simulink model "test1"  (R2018a)
settings: Solver=VariableStepAuto  StartTime=0.0  StopTime=4000  FixedStep=0.01  RelTol=1e-3
InitFcn:
  | run constants
StopFcn:
  | run runafter
values from neighbouring files (symbols this model uses):
  F_0 = [0 0 0]    [constants2.m]
  F_grav = mass_0 * g_h    (= 7.95745129095)    [constants2.m]
  phi_noise = noise_att_on * noise_att_mag    [constants2.m]
  pm_0 = [0 0 0]    [constants2.m]
  Psi_noise = noise_att_on * noise_att_mag    [constants2.m]
  T_d = Td_on * [0.001 0.001 0.001]    [constants2.m]
  theta_noise = noise_att_on * noise_att_mag    [constants2.m]
  Vm_0 = [0 Vc 0]    [constants2.m]
  xme_0 = [1 2 3]    [constants2.m]
libraries: shared6dof x6, simulink x4, shared6dofsys x3, sharedutil x1, dspmathops x1
CloseFcn:
  | run runafter
settings Model: EnablePacing=on  PacingRate=1000  Creator=Matt  LastModifiedBy=matth

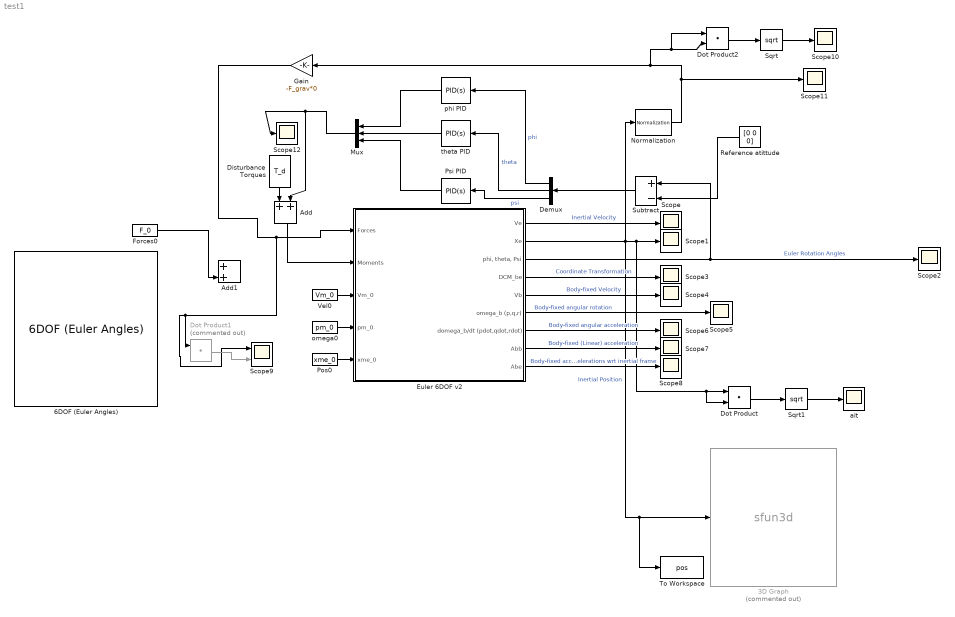
== system test1 ==
  3D Graph : S-Function  Commented=on  LoadFcn=if exist('sfun3d','file'), sfun3d([],[],[],'LoadBlock'); end  FunctionName=sfun3d  Parameters=ax,T,np,cp,gd,ls,mk,mx,hd,tb  SFunctionDeploymentMode=off  EnableBusSupport=off  mask(3D Graph){np=1, ax=[-3 3 -3 3 -3 3], mx=1e4, T=0.1, cp=[3 2 1], gd=on, hd=off, tb=off, ls=-, mk=none}
      mask prompts: np "Number of moving points (lines)"; ax "Range: [xmin xmax  ymin ymax zmin zmax]"; mx "Max number of points in each line"; T "Sampling Time"; cp "Camera position (use [0 0 1] for 2D XY view)"; gd "Grid (on|off)"; hd "HeadMarkers (on|off)"; tb "Toolbar (on|off)"; ls "LineStyle"; mk "LineMarker"
      mask help:
      | This block plots the position of several points in the XYZ space. The input contains the coordinates of all the points (x1,y1,z1,x2,y2,z2,...).
      | The number of moving points (lines), the XYZ ranges, sampling time, camera position, and grid (among other things) can be set as mask parameters.
      settings: CopyFcn=if exist('sfun3d','file'), sfun3d([],[],[],'CopyBlock'); end  DeleteFcn=if exist('sfun3d','file'), sfun3d([],[],[],'DeleteBlock'); end  NameChangeFcn=if exist('sfun3d','file'), sfun3d([],[],[],'NameChange'); end
      mask Help:
      | This block plots the position of several points in the XYZ space. The input contains the coordinates of all the points (x1,y1,z1,x2,y2,z2,...).
      | The number of moving points (lines), the XYZ ranges, sampling time, camera position, and grid (among other things) can be set as mask parameters.
      mask TypeOptions ls: - | -- | : | -. | none
      mask TypeOptions mk: none | . | + | o | * | x | square | diamond | v | ^ | > | < | pentagram | hexagram
      mask Display: plot([.05 .95 .95 .05 .05],[.45 .45 .95 .95 .45], 0.5+cos(0:0.1:2*pi)*0.3,0.7+sin(0:0.1:2*pi)*0.2)
  6DOF (Euler Angles) : shared6dof/6DOF (Euler Angles)  units=Metric (MKS)  mtype=Fixed  rep=Euler Angles  xme_0=[0 0 0]  Vm_0=[0 0 0]  eul_0=[0 0 0]  pm_0=[0 0 0]  mass_0=1.0  mass_e=0.5  mass_f=2.0  inertia=eye(3)  inertia_e=eye(3)  inertia_f=2*eye(3)  k_quat=1.0  vre_flag=on  abi_flag=off  aMode=0
      settings: SourceProductBaseCode=AE
  Add : Sum
  Add1 : Sum
  Demux : Demux  Outputs=3
  Disturbance Torques : Constant  Value=T_d
  Dot Product : DotProduct  InputSameDT=on  OutDataTypeStr=Inherit: Inherit via internal rule
  Dot Product1 : DotProduct  Commented=on  InputSameDT=on  OutDataTypeStr=Inherit: Inherit via internal rule
  Dot Product2 : DotProduct  InputSameDT=on  OutDataTypeStr=Inherit: Inherit via internal rule
  Euler 6DOF v2 : Subsystem
  Forces0 : Constant  Value=F_0
  Gain : Gain  Gain=-F_grav*0
  Mux : Mux  Inputs=3
  Normalization : dspmathops/Normalization  NormType=2-norm  Bias=1e-10  NormOver=Each column  Dimension=1  roundingMode=Floor  overflowMode=off  accumDataTypeStr=Inherit: Same as product output  accumLastDataTypeStr=Inherit: Same as product output  outputDataTypeStr=Inherit: Same as product output  outputMin=[]  outputMax=[]  outputLastDataTypeStr=Inherit: Same as product output
      settings: SourceProductName=DSP System Toolbox
  Pos0 : Constant  Value=xme_0
  Psi PID : simulink/Continuous/PID Controller  Controller=PID  TimeDomain=Continuous-time  SampleTime=-1  IntegratorMethod=Forward Euler  FilterMethod=Forward Euler  Form=Parallel  UseFilter=on  ControllerParametersSource=internal  P=-730.157338378478  I=-36.609264068618  D=-2842.71233291057  N=10.4897155810233  InitialConditionSource=internal  InitialConditionForIntegrator=0  InitialConditionForFilter=0  ExternalReset=none  LimitOutput=off  UpperSaturationLimit=inf  LowerSaturationLimit=-inf  LinearizeAsGain=on  AntiWindupMode=none  Kb=1  TrackingMode=off  Kt=1  PParamMin=[]  PParamMax=[]  IParamMin=[]  IParamMax=[]  DParamMin=[]  DParamMax=[]  NParamMin=[]  NParamMax=[]  KbParamMin=[]  KbParamMax=[]  KtParamMin=[]  KtParamMax=[]  POutMin=[]  POutMax=[]  IOutMin=[]  IOutMax=[]  DOutMin=[]  DOutMax=[]  NOutMin=[]  NOutMax=[]  KbOutMin=[]  KbOutMax=[]  KtOutMin=[]  KtOutMax=[]  IntegratorOutMin=[]  IntegratorOutMax=[]  FilterOutMin=[]  FilterOutMax=[]  SumOutMin=[]  SumOutMax=[]  SumI1OutMin=[]  SumI1OutMax=[]  SumI2OutMin=[]  SumI2OutMax=[]  SumI3OutMin=[]  SumI3OutMax=[]  SumDOutMin=[]  SumDOutMax=[]  SaturationOutMin=[]  SaturationOutMax=[]  IntegratorContinuousStateAttributes=''  IntegratorStateMustResolveToSignalObject=off  IntegratorRTWStateStorageClass=Auto  FilterContinuousStateAttributes=''  FilterStateMustResolveToSignalObject=off  FilterRTWStateStorageClass=Auto  DifferentiatorICPrevScaledInput=0  DifferentiatorOutMin=[]  DifferentiatorOutMax=[]  FilterDiffOutCoefMin=[]  FilterDiffOutCoefMax=[]  SumDenOutMin=[]  SumDenOutMax=[]  SumNumOutMin=[]  SumNumOutMax=[]  ReciprocalOutMin=[]  ReciprocalOutMax=[]  DivideOutMin=[]  DivideOutMax=[]  TunerSelectOption=Transfer Function Based (PID Tuner App)
  Reference atittude : Constant  Value=[0 0 0]
  Scope{,1..8,10..12} (12 alike) : Scope
  Scope9 : Scope  NumInputPorts=2
  Sqrt : Sqrt  SaturateOnIntegerOverflow=on
  Sqrt1 : Sqrt  SaturateOnIntegerOverflow=on
  Subtract : Sum  Inputs=+-
  To Workspace : ToWorkspace  VariableName=pos  SaveFormat=Timeseries  SampleTime=-1
  Vel0 : Constant  Value=Vm_0
  alt : Scope
  "omega0 " : Constant  Value=pm_0
  "phi PID " : simulink/Continuous/PID Controller  Controller=PID  TimeDomain=Continuous-time  SampleTime=-1  IntegratorMethod=Forward Euler  FilterMethod=Forward Euler  Form=Parallel  UseFilter=on  ControllerParametersSource=internal  P=-464.198158177747  I=-21.7313338529705  D=-2434.80245399495  N=5.45397025421619  InitialConditionSource=internal  InitialConditionForIntegrator=0  InitialConditionForFilter=0  ExternalReset=none  LimitOutput=off  UpperSaturationLimit=inf  LowerSaturationLimit=-inf  LinearizeAsGain=on  AntiWindupMode=none  Kb=1  TrackingMode=off  Kt=1  PParamMin=[]  PParamMax=[]  IParamMin=[]  IParamMax=[]  DParamMin=[]  DParamMax=[]  NParamMin=[]  NParamMax=[]  KbParamMin=[]  KbParamMax=[]  KtParamMin=[]  KtParamMax=[]  POutMin=[]  POutMax=[]  IOutMin=[]  IOutMax=[]  DOutMin=[]  DOutMax=[]  NOutMin=[]  NOutMax=[]  KbOutMin=[]  KbOutMax=[]  KtOutMin=[]  KtOutMax=[]  IntegratorOutMin=[]  IntegratorOutMax=[]  FilterOutMin=[]  FilterOutMax=[]  SumOutMin=[]  SumOutMax=[]  SumI1OutMin=[]  SumI1OutMax=[]  SumI2OutMin=[]  SumI2OutMax=[]  SumI3OutMin=[]  SumI3OutMax=[]  SumDOutMin=[]  SumDOutMax=[]  SaturationOutMin=[]  SaturationOutMax=[]  IntegratorContinuousStateAttributes=''  IntegratorStateMustResolveToSignalObject=off  IntegratorRTWStateStorageClass=Auto  FilterContinuousStateAttributes=''  FilterStateMustResolveToSignalObject=off  FilterRTWStateStorageClass=Auto  DifferentiatorICPrevScaledInput=0  DifferentiatorOutMin=[]  DifferentiatorOutMax=[]  FilterDiffOutCoefMin=[]  FilterDiffOutCoefMax=[]  SumDenOutMin=[]  SumDenOutMax=[]  SumNumOutMin=[]  SumNumOutMax=[]  ReciprocalOutMin=[]  ReciprocalOutMax=[]  DivideOutMin=[]  DivideOutMax=[]  TunerSelectOption=Transfer Function Based (PID Tuner App)
  theta PID : simulink/Continuous/PID Controller  Controller=PID  TimeDomain=Continuous-time  SampleTime=-1  IntegratorMethod=Forward Euler  FilterMethod=Forward Euler  Form=Parallel  UseFilter=on  ControllerParametersSource=internal  P=-568.423410964435  I=-28.5001924417647  D=-2213.03320065217  N=10.4897155810233  InitialConditionSource=internal  InitialConditionForIntegrator=0  InitialConditionForFilter=0  ExternalReset=none  LimitOutput=off  UpperSaturationLimit=inf  LowerSaturationLimit=-inf  LinearizeAsGain=on  AntiWindupMode=none  Kb=1  TrackingMode=off  Kt=1  PParamMin=[]  PParamMax=[]  IParamMin=[]  IParamMax=[]  DParamMin=[]  DParamMax=[]  NParamMin=[]  NParamMax=[]  KbParamMin=[]  KbParamMax=[]  KtParamMin=[]  KtParamMax=[]  POutMin=[]  POutMax=[]  IOutMin=[]  IOutMax=[]  DOutMin=[]  DOutMax=[]  NOutMin=[]  NOutMax=[]  KbOutMin=[]  KbOutMax=[]  KtOutMin=[]  KtOutMax=[]  IntegratorOutMin=[]  IntegratorOutMax=[]  FilterOutMin=[]  FilterOutMax=[]  SumOutMin=[]  SumOutMax=[]  SumI1OutMin=[]  SumI1OutMax=[]  SumI2OutMin=[]  SumI2OutMax=[]  SumI3OutMin=[]  SumI3OutMax=[]  SumDOutMin=[]  SumDOutMax=[]  SaturationOutMin=[]  SaturationOutMax=[]  IntegratorContinuousStateAttributes=''  IntegratorStateMustResolveToSignalObject=off  IntegratorRTWStateStorageClass=Auto  FilterContinuousStateAttributes=''  FilterStateMustResolveToSignalObject=off  FilterRTWStateStorageClass=Auto  DifferentiatorICPrevScaledInput=0  DifferentiatorOutMin=[]  DifferentiatorOutMax=[]  FilterDiffOutCoefMin=[]  FilterDiffOutCoefMax=[]  SumDenOutMin=[]  SumDenOutMax=[]  SumNumOutMin=[]  SumNumOutMax=[]  ReciprocalOutMin=[]  ReciprocalOutMax=[]  DivideOutMin=[]  DivideOutMax=[]  TunerSelectOption=Transfer Function Based (PID Tuner App)
  wires:
  Euler 6DOF v2/1(Ve) -> Scope/1  "Inertial Velocity"
  Euler 6DOF v2/2(Xe) -> Dot Product/2, Dot Product/1, Scope1/1, Normalization/1, To Workspace/1, 3D Graph/1  "Inertial Position"
  Euler 6DOF v2/3("phi, theta, Psi") -> Subtract/1, Scope2/1  "Euler Rotation Angles"
  Euler 6DOF v2/4(DCM_be) -> Scope3/1  "Coordinate Transformation"
  Euler 6DOF v2/5(Vb) -> Scope4/1  "Body-fixed Velocity"
  Euler 6DOF v2/6(omega_b (p,q,r)) -> Scope5/1  "Body-fixed angular rotation"
  Euler 6DOF v2/7(domega_b/dt (pdot,qdot,rdot)) -> Scope6/1  "Body-fixed angular acceleration"
  Euler 6DOF v2/8(Abb) -> Scope7/1  "Body-fixed (Linear) acceleration"
  Euler 6DOF v2/9(Abe) -> Scope8/1  "Body-fixed accelerations wrt inertial frame"
  Reference atittude/1 -> Subtract/2
  Demux/1 -> "phi PID "/1  "phi"
  Demux/2 -> theta PID/1  "theta"
  Demux/3 -> Psi PID/1  "psi"
  "phi PID "/1 -> Mux/1
  theta PID/1 -> Mux/2
  Psi PID/1 -> Mux/3
  Mux/1 -> Add/2, Scope12/1
  Subtract/1 -> Demux/1
  Forces0/1 -> Add1/2
  Vel0/1 -> Euler 6DOF v2/3(Vm_0)
  Pos0/1 -> Euler 6DOF v2/5("xme_0 ")
  "omega0 "/1 -> Euler 6DOF v2/4("pm_0 ")
  Disturbance Torques/1 -> Add/1
  Add/1 -> Euler 6DOF v2/2(Moments)
  Normalization/1 -> Scope11/1, Dot Product2/2, Dot Product2/1, Gain/1
  Gain/1 -> Scope9/1, Dot Product1/1, Euler 6DOF v2/1(Forces)
  Dot Product1/1 -> Scope9/2
  Dot Product2/1 -> Sqrt/1
  Sqrt/1 -> Scope10/1
  Dot Product/1 -> Sqrt1/1
  Sqrt1/1 -> alt/1

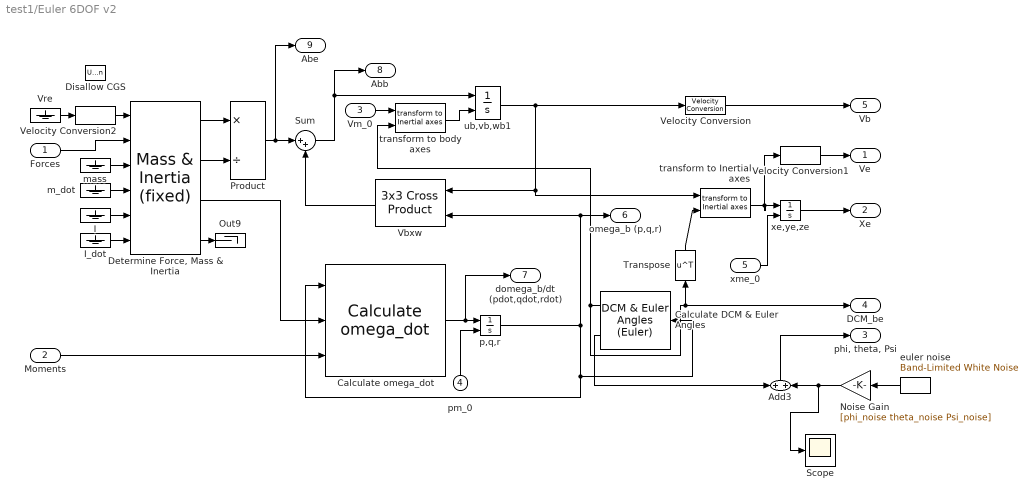
== system test1/Euler 6DOF v2 ==
  Forces : Inport  Unit=N  PortDimensions=3
  Moments : Inport  Port=2  Unit=N*m  PortDimensions=3
  Vm_0 : Inport  Port=3
  "pm_0 " : Inport  Port=4
  "xme_0 " : Inport  Port=5
  Add3 : Sum
  Calculate DCM & Euler Angles : shared6dofsys/DCM & Euler Angles (Euler)  aMode=aMode
      settings: SourceProductName=Aerospace Blockset  SourceProductBaseCode=AE
  Calculate omega_dot : shared6dofsys/Calculate omega_dot  aMode=aMode
      settings: SourceProductName=Aerospace Blockset  SourceProductBaseCode=AE
  "Determine Force, Mass & Inertia" : shared6dofsys/Mass & Inertia (fixed)  aMode=aMode
      settings: SourceProductName=Aerospace Blockset  SourceProductBaseCode=AE
  Disallow CGS : UnitConfiguration  UnitSystemsStr=English,SI,SI (extended)  AllowAllUnitSystems=off
  I : Ground
  I_dot : Ground
  Noise Gain : Gain  Gain=[phi_noise theta_noise Psi_noise]
  Out9 : Terminator
  Product : Product  Inputs=*/  SaturateOnIntegerOverflow=on  OutDataTypeStr=Inherit: Same as first input
  Scope : Scope
  Sum : Sum  Inputs=|++  SaturateOnIntegerOverflow=on
  Transpose : Math  Operator=transpose  SaturateOnIntegerOverflow=on
  Vbxw : sharedutil/3x3 Cross Product  aMode=aMode
      settings: SourceProductBaseCode=AE
  Velocity Conversion : shared6dof/6DOF (Euler Angles)/Velocity Conversion
      settings: SourceProductName=Aerospace Blockset  SourceProductBaseCode=AE
  Velocity Conversion1 : shared6dof/6DOF (Euler Angles)/Velocity Conversion1
      settings: SourceProductName=Aerospace Blockset  SourceProductBaseCode=AE
  Velocity Conversion2 : shared6dof/6DOF (Euler Angles)/Velocity Conversion2
      settings: SourceProductName=Aerospace Blockset  SourceProductBaseCode=AE
  Vre : Ground
  euler noise : simulink/Sources/Band-Limited White Noise  Cov=[0.1]  Ts=1  seed=[23341]
  m_dot : Ground
  mass : Ground
  "p,q,r " : Integrator  InitialConditionSource=external  InitialCondition=pm_0
  "transform to Inertial axes " : shared6dof/6DOF (Euler Angles)/transform to Inertial axes   SystemSampleTime=-1
      settings: SourceProductName=Aerospace Blockset  SourceProductBaseCode=AE
  transform to body axes : shared6dof/6DOF (Euler Angles)/transform to Inertial axes   SystemSampleTime=-1
      settings: SourceProductName=Aerospace Blockset  SourceProductBaseCode=AE
  ub,vb,wb1 : Integrator  InitialConditionSource=external  InitialCondition=Vm_0
  xe,ye,ze : Integrator  InitialConditionSource=external  InitialCondition=xme_0
  Ve : Outport  Unit=m/s
  Xe : Outport  Port=2  Unit=m
  "phi, theta, Psi" : Outport  Port=3  Unit=rad
  DCM_be : Outport  Port=4  Unit=1
  Vb : Outport  Port=5  Unit=m/s
  omega_b (p,q,r) : Outport  Port=6  Unit=rad/s
  domega_b/dt (pdot,qdot,rdot) : Outport  Port=7  Unit=rad/s^2
  Abb : Outport  Port=8  Unit=m/s^2
  Abe : Outport  Port=9  Unit=m/s^2
  wires:
  Calculate DCM & Euler Angles/1 -> transform to body axes/2, Transpose/1, DCM_be/1
  Vbxw/1 -> Sum/2
  Velocity Conversion/1 -> Vb/1
  xe,ye,ze/1 -> Xe/1
  Vre/1 -> Velocity Conversion2/1
  Calculate DCM & Euler Angles/2 -> Add3/1
  "p,q,r "/1 -> Calculate omega_dot/1, Calculate DCM & Euler Angles/1, omega_b (p,q,r)/1, Vbxw/2
  Product/1 -> Sum/1, Abe/1
  Moments/1 -> Calculate omega_dot/3
  "Determine Force, Mass & Inertia"/2 -> Product/2
  "transform to Inertial axes "/1 -> xe,ye,ze/1, Velocity Conversion1/1
  "Determine Force, Mass & Inertia"/4 -> Out9/1
  Transpose/1 -> "transform to Inertial axes "/2
  mass/1 -> "Determine Force, Mass & Inertia"/3
  Velocity Conversion1/1 -> Ve/1
  Calculate omega_dot/1 -> "p,q,r "/1, domega_b/dt (pdot,qdot,rdot)/1
  I/1 -> "Determine Force, Mass & Inertia"/5
  "Determine Force, Mass & Inertia"/3 -> Calculate omega_dot/2
  ub,vb,wb1/1 -> "transform to Inertial axes "/1, Vbxw/1, Velocity Conversion/1
  "Determine Force, Mass & Inertia"/1 -> Product/1
  Forces/1 -> "Determine Force, Mass & Inertia"/2
  Velocity Conversion2/1 -> "Determine Force, Mass & Inertia"/1
  I_dot/1 -> "Determine Force, Mass & Inertia"/6
  Sum/1 -> Abb/1, ub,vb,wb1/1
  m_dot/1 -> "Determine Force, Mass & Inertia"/4
  Vm_0/1 -> transform to body axes/1
  "pm_0 "/1 -> "p,q,r "/2
  "xme_0 "/1 -> xe,ye,ze/2
  Noise Gain/1 -> Scope/1, Add3/2
  Add3/1 -> "phi, theta, Psi"/1
  euler noise/1 -> Noise Gain/1
  transform to body axes/1 -> ub,vb,wb1/2
